simulink model "task4"  (R2024a)
settings: Solver=FixedStepAuto  StartTime=0.0  StopTime=10.0  FixedStep=0.001  MaxStep=0.1  RelTol=1e-20
undefined symbols (not defined in the file): A, B, C, D, G, K, N_inv, Q, x0, Y, z0_hat
settings Model: Creator=sizgr  LastModifiedBy=sizgr

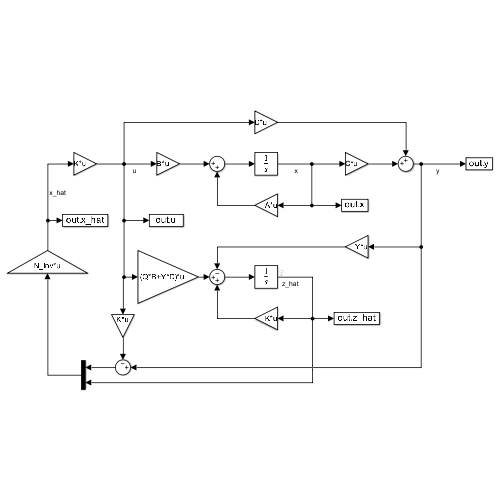
[thumbnail: Simulink's stored preview of the top-level diagram]
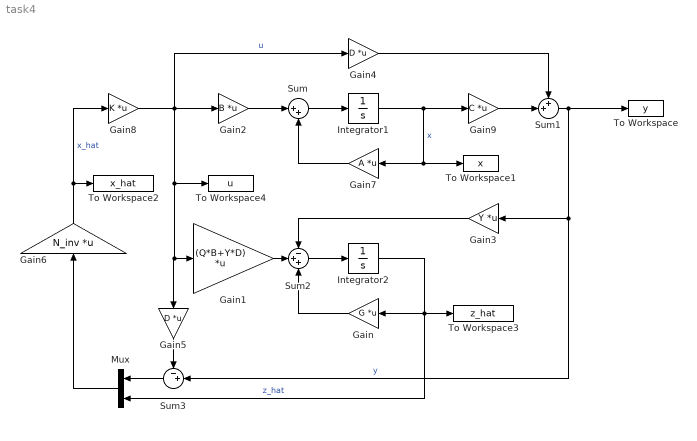
== system task4 ==
  Gain : Gain  Gain=G  Multiplication=Matrix(K*u)
  Gain1 : Gain  Gain=(Q*B+Y*D)  Multiplication=Matrix(K*u)
  Gain2 : Gain  Gain=B  Multiplication=Matrix(K*u)
  Gain3 : Gain  Gain=Y  Multiplication=Matrix(K*u)
  Gain4 : Gain  Gain=D  Multiplication=Matrix(K*u)
  Gain5 : Gain  Gain=D  Multiplication=Matrix(K*u)
  Gain6 : Gain  Gain=N_inv  Multiplication=Matrix(K*u)
  Gain7 : Gain  Gain=A  Multiplication=Matrix(K*u)
  Gain8 : Gain  Gain=K  Multiplication=Matrix(K*u)
  Gain9 : Gain  Gain=C  Multiplication=Matrix(K*u)
  Integrator1 : Integrator  InitialCondition=x0
  Integrator2 : Integrator  InitialCondition=z0_hat
  Mux : Mux  Inputs=2
  Sum : Sum  Inputs=|++
  Sum1 : Sum  Inputs=++|
  Sum2 : Sum  Inputs=-++
  Sum3 : Sum  Inputs=-+|
  To Workspace : ToWorkspace  VariableName=y  SaveFormat=Timeseries  SampleTime=-1
  To Workspace1 : ToWorkspace  VariableName=x  SaveFormat=Timeseries  SampleTime=-1
  To Workspace2 : ToWorkspace  VariableName=x_hat  SaveFormat=Timeseries  SampleTime=-1
  To Workspace3 : ToWorkspace  VariableName=z_hat  SaveFormat=Timeseries  SampleTime=-1
  To Workspace4 : ToWorkspace  VariableName=u  SaveFormat=Timeseries  SampleTime=-1
  wires:
  Gain6/1 -> To Workspace2/1, Gain8/1  "x_hat"
  Integrator1/1 -> To Workspace1/1, Gain7/1, Gain9/1  "x"
  Gain8/1 -> Gain2/1, Gain4/1, To Workspace4/1, Gain5/1, Gain1/1  "u"
  Gain2/1 -> Sum/1
  Sum/1 -> Integrator1/1
  Gain7/1 -> Sum/2
  Gain9/1 -> Sum1/2
  Gain4/1 -> Sum1/1
  Sum1/1 -> Sum3/2, Gain3/1, To Workspace/1  "y"
  Integrator2/1 -> To Workspace3/1, Mux/2, Gain/1  "z_hat"
  Sum2/1 -> Integrator2/1
  Gain/1 -> Sum2/3
  Gain1/1 -> Sum2/2
  Gain3/1 -> Sum2/1
  Gain5/1 -> Sum3/1
  Sum3/1 -> Mux/1
  Mux/1 -> Gain6/1
